simulink model "untitled1"  (R2016b)
settings: Solver=VariableStepAuto  StartTime=0.0  StopTime=10.0  RelTol=1e-3
settings Model: Creator=lenovo  LastModifiedBy=lenovo

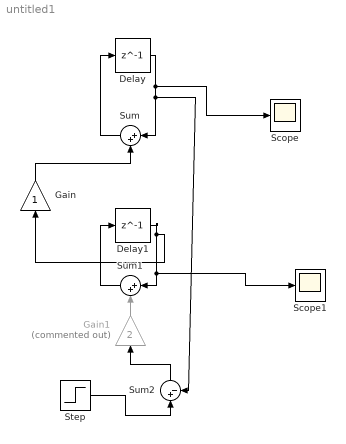
== system untitled1 ==
  Delay : Delay  DelayLength=1
  Delay1 : Delay  DelayLength=1
  Gain : Gain
  Gain1 : Gain  Commented=on  Gain=2
  Scope : Scope
  Scope1 : Scope
  Step : Step  SampleTime=0
  Sum : Sum  Inputs=|++
  Sum1 : Sum  Inputs=|++
  Sum2 : Sum  Inputs=|+-
  wires:
  Delay1/1 -> Gain/1, Scope1/1, Sum1/1
  Sum/1 -> Delay/1
  Delay/1 -> Scope/1, Sum2/2, Sum/1
  Sum1/1 -> Delay1/1
  Sum2/1 -> Gain1/1
  Step/1 -> Sum2/1
  Gain/1 -> Sum/2
  Gain1/1 -> Sum1/2
